simulink model "dynamic_8_edit"  (R2020b)
settings: Solver=ode5  StartTime=0.0  StopTime=60  FixedStep=0.1  RelTol=1e-3
libraries: simulink x2
settings Model: Creator=skets  LastModifiedBy=skets
settings SolverCC: ConcurrentTasks=on  PositivePriorityOrder=on
settings DataIOCC: ReturnWorkspaceOutputs=off
settings OptimizationCC: BlockReduction=off  DefaultParameterBehavior=Inlined  EnhancedBackFolding=on  PassReuseOutputArgsThreshold=0  OptimizeBlockOrder=speed  DifferentSizesBufferReuse=on  OptimizationCustomize=off
settings DebuggingCC: ParameterTunabilityLossMsg=error  ArithmeticOperatorsInVariantConditions=warning
settings SFSimCC: SimUseLocalCustomCode=off  MATLABDynamicMemAlloc=off  CustomCodeUndefinedFunction=UseInterfaceOnly
settings RTWCC: PackageGeneratedCodeAndArtifacts=on  PackageName=dynamic_circle  RTWUseLocalCustomCode=off  Toolchain=MinGW64 | gmake (64-bit Windows)  BuildConfiguration=Debug
settings CodeAppCC: ForceParamTrailComments=on  OperatorAnnotations=on

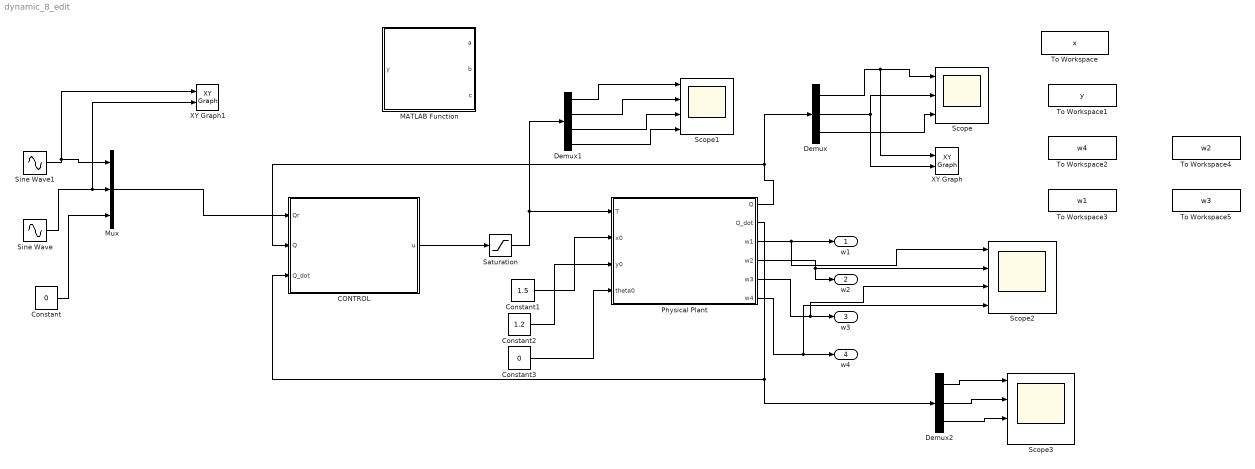
== system dynamic_8_edit ==
  CONTROL : Subsystem
  Constant : Constant  Value=0
  Constant1 : Constant  Value=1.5
  Constant2 : Constant  Value=1.2
  Constant3 : Constant  Value=0
  Demux : Demux  Outputs=3
  Demux1 : Demux
  Demux2 : Demux  Outputs=3
  MATLAB Function : MATLAB Function  TreatAsAtomicUnit=on
  Mux : Mux  Inputs=3
  Physical Plant : Subsystem
  Saturation : Saturate  UpperLimit=5  LowerLimit=-5
  Scope : Scope  NumInputPorts=3
  Scope1 : Scope  NumInputPorts=4
  Scope2 : Scope  NumInputPorts=4
  Scope3 : Scope  NumInputPorts=4
  Sine Wave : Sin  Bias=1.2  Frequency=4*pi/30
  Sine Wave1 : Sin  Bias=1.5  Frequency=2*pi/30
  To Workspace : ToWorkspace  VariableName=x  SampleTime=-1
  To Workspace1 : ToWorkspace  VariableName=y  SampleTime=-1
  To Workspace2 : ToWorkspace  VariableName=w4  SampleTime=-1
  To Workspace3 : ToWorkspace  VariableName=w1  SampleTime=-1
  To Workspace4 : ToWorkspace  VariableName=w2  SampleTime=-1
  To Workspace5 : ToWorkspace  VariableName=w3  SampleTime=-1
  XY Graph : simulink/Sinks/XY Graph  xmin=0  xmax=3  ymin=0  ymax=3  st=-1
  XY Graph1 : simulink/Sinks/XY Graph  xmin=0  xmax=2  ymin=0  ymax=2  st=-1
  w1 : Outport  VectorParamsAs1DForOutWhenUnconnected=off
  w2 : Outport  Port=2  VectorParamsAs1DForOutWhenUnconnected=off
  w3 : Outport  Port=3  VectorParamsAs1DForOutWhenUnconnected=off
  w4 : Outport  Port=4  VectorParamsAs1DForOutWhenUnconnected=off
  wires:
  Sine Wave/1 -> XY Graph1/2, Mux/2
  Constant/1 -> Mux/3
  Sine Wave1/1 -> XY Graph1/1, Mux/1
  Mux/1 -> CONTROL/1(Qr)
  CONTROL/1(u) -> Saturation/1
  Saturation/1 -> Demux1/1, Physical Plant/1(T)
  Physical Plant/3(w1) -> Scope2/1, w1/1
  Physical Plant/4(w2) -> Scope2/2, w2/1
  Physical Plant/5(w3) -> Scope2/3, w3/1
  Demux/1 -> XY Graph/1, Scope/1
  Demux/2 -> Scope/2, XY Graph/2
  Demux/3 -> Scope/3
  Demux1/1 -> Scope1/1
  Demux1/2 -> Scope1/2
  Demux1/3 -> Scope1/3
  Demux1/4 -> Scope1/4
  Physical Plant/2(Q_dot) -> CONTROL/3(Q_dot), Demux2/1
  Demux2/1 -> Scope3/1
  Demux2/2 -> Scope3/2
  Demux2/3 -> Scope3/3
  Constant1/1 -> Physical Plant/2(x0)
  Constant2/1 -> Physical Plant/3(y0)
  Constant3/1 -> Physical Plant/4(theta0)
  Physical Plant/6(w4) -> Scope2/4, w4/1
  Physical Plant/1(Q) -> CONTROL/2(Q), Demux/1

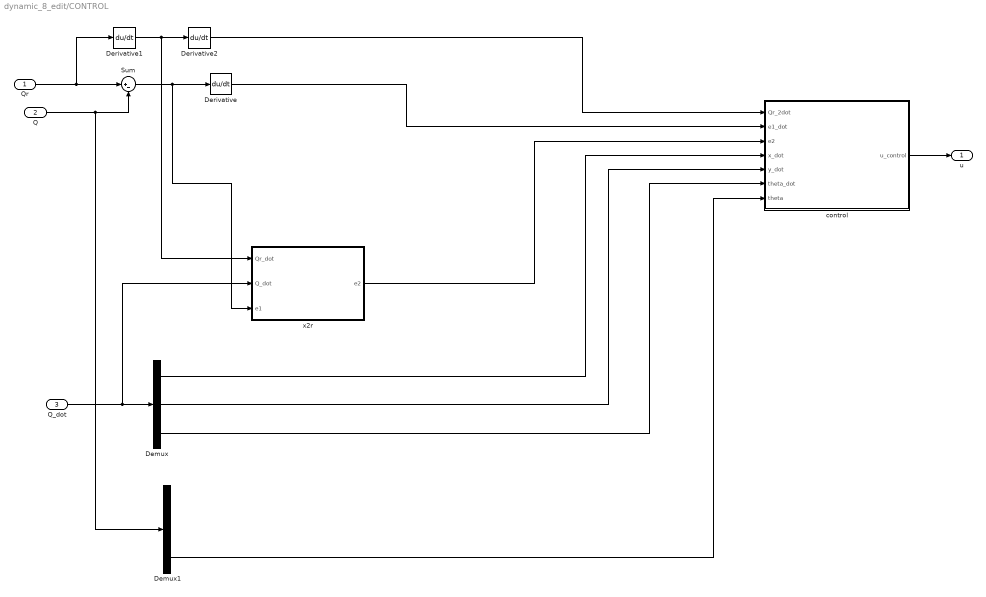
== system dynamic_8_edit/CONTROL ==
  Qr : Inport
  Q : Inport  Port=2  PortDimensions=3
  Q_dot : Inport  Port=3
  Demux : Demux  Outputs=3
  Demux1 : Demux  Outputs=3
  Derivative : Derivative
  Derivative1 : Derivative
  Derivative2 : Derivative
  Sum : Sum  Inputs=|+-
  control : MATLAB Function  TreatAsAtomicUnit=on
  x2r : MATLAB Function  TreatAsAtomicUnit=on
  u : Outport  VectorParamsAs1DForOutWhenUnconnected=off
  wires:
  Qr/1 -> Derivative1/1, Sum/1
  control/1(u_control) -> u/1
  Q/1 -> Demux1/1, Sum/2
  Demux/1 -> control/4(x_dot)
  Demux/2 -> control/5(y_dot)
  Demux/3 -> control/6(theta_dot)
  Demux1/3 -> control/7(theta)
  Sum/1 -> x2r/3(e1), Derivative/1
  Derivative2/1 -> control/1(Qr_2dot)
  Derivative/1 -> control/2(e1_dot)
  x2r/1(e2) -> control/3(e2)
  Derivative1/1 -> x2r/1(Qr_dot), Derivative2/1
  Q_dot/1 -> x2r/2(Q_dot), Demux/1

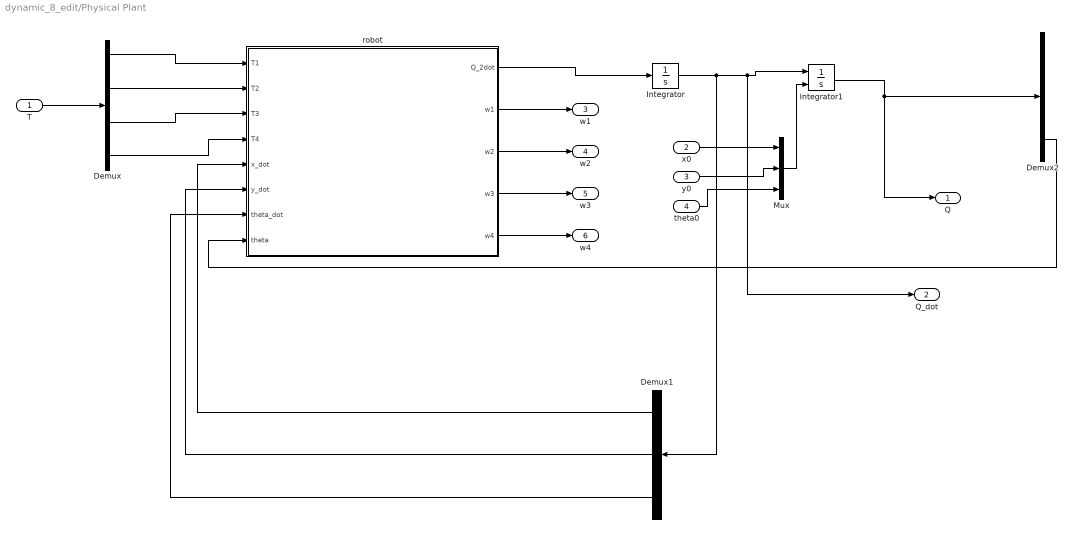
== system dynamic_8_edit/Physical Plant ==
  T : Inport  PortDimensions=4
  x0 : Inport  Port=2  PortDimensions=1
  y0 : Inport  Port=3  PortDimensions=1
  theta0 : Inport  Port=4  PortDimensions=1
  Demux : Demux
  Demux1 : Demux  Outputs=3
  Demux2 : Demux  Outputs=3
  Integrator : Integrator
  Integrator1 : Integrator  InitialConditionSource=external  InitialCondition=[0.5 1 0]
  Mux : Mux  Inputs=3
  robot : MATLAB Function  TreatAsAtomicUnit=on
  Q : Outport  VectorParamsAs1DForOutWhenUnconnected=off
  Q_dot : Outport  Port=2  VectorParamsAs1DForOutWhenUnconnected=off
  w1 : Outport  Port=3  VectorParamsAs1DForOutWhenUnconnected=off
  w2 : Outport  Port=4  VectorParamsAs1DForOutWhenUnconnected=off
  w3 : Outport  Port=5  VectorParamsAs1DForOutWhenUnconnected=off
  w4 : Outport  Port=6  VectorParamsAs1DForOutWhenUnconnected=off
  wires:
  Demux/1 -> robot/1(T1)
  Demux/2 -> robot/2(T2)
  Demux/3 -> robot/3(T3)
  Demux/4 -> robot/4(T4)
  robot/1(Q_2dot) -> Integrator/1
  Demux1/1 -> robot/5(x_dot)
  Demux1/2 -> robot/6(y_dot)
  Demux1/3 -> robot/7(theta_dot)
  Integrator1/1 -> Demux2/1, Q/1
  Demux2/3 -> robot/8(theta)
  T/1 -> Demux/1
  robot/2(w1) -> w1/1
  robot/3(w2) -> w2/1
  robot/4(w3) -> w3/1
  robot/5(w4) -> w4/1
  Integrator/1 -> Demux1/1, Integrator1/1, Q_dot/1
  Mux/1 -> Integrator1/2
  x0/1 -> Mux/1
  y0/1 -> Mux/2
  theta0/1 -> Mux/3

== matlab function dynamic_8_edit/Physical Plant/robot ==
  data: T1 input; Q_2dot output; T2 input; T3 input; T4 input; x_dot input; y_dot input; theta_dot input; theta input; w1 output; w2 output; w3 output; w4 output
function [Q_2dot,w1,w2,w3,w4]  = fcn(T1, T2, T3, T4,x_dot,y_dot,theta_dot,theta)

m=5;
I=5;
Ib=0.1;
l1= 0.3;
l2=0.3;
r=0.048;
g=9.8;
u=0.01;
N = m*g/4;
M=[(m+4*Ib/(r*r)) 0 0; 0 (m+4*Ib/(r*r)) 0; 0 0 (I+4*Ib*(l1+l2)*(l1+l2)/(r*r))];
C= [(m+4*Ib/(r*r))*y_dot*theta_dot;-(m+4*Ib/(r*r))*x_dot*theta_dot;0 ];
B=(1/r)*[(cos(theta)+sin(theta)) (cos(theta)-sin(theta)) (cos(theta)+sin(theta)) (cos(theta)-sin(theta));
         (-cos(theta)+sin(theta)) (cos(theta)+sin(theta)) (-cos(theta)+sin(theta)) (cos(theta)+sin(theta)); 
         (-(l1+l2)) (l1+l2) (l1+l2) (-(l1+l2)) ];
T=[T1;T2;T3;T4];
xm= cos(theta)*x_dot+sin(theta)*y_dot;
ym= -sin(theta)*x_dot+cos(theta)*y_dot;
w1 = (1/r)*(xm-ym-(l1+l2)*theta_dot);
w2 = (1/r)*(xm+ym+(l1+l2)*theta_dot);
w3 = (1/r)*(xm-ym+(l1+l2)*theta_dot);
w4 = (1/r)*(xm+ym-(l1+l2)*theta_dot);
w_max = 2;
if w1 > w_max
    w1 = w_max; %w = 20.83
elseif w1 < -w_max
    w1 = -w_max;
end
if w2 > w_max
    w2 = w_max;
elseif w2 < -w_max
    w2 = -w_max;
end
if w3 > w_max
    w3 = w_max;
elseif w3 < -w_max
    w3 = -w_max;
end
if w4 > w_max
    w4 = w_max;
elseif w4 < -w_max
    w4 = -w_max;
end
Xi=[u*r*N*sign(w1);u*r*N*sign(w2);u*r*N*sign(w3);u*N*r*sign(w4)];

Q_2dot=inv(M)*(B*T-C-B*Xi);

== matlab function dynamic_8_edit/CONTROL/control ==
  data: Qr_2dot input; u_control output; e1_dot input; e2 input; x_dot input; y_dot input; theta_dot input; theta input
function u_control = fcn(Qr_2dot,e1_dot,e2,x_dot,y_dot,theta_dot,theta)

m=5;
I=5;
Ib=0.1;
l1= 0.3;
l2=0.3;
r=0.048;
g=9.8;
u=0.01;
N = m*g/4;
M=[(m+4*Ib/(r*r)) 0 0; 0 (m+4*Ib/(r*r)) 0; 0 0 (I+4*Ib*(l1+l2)*(l1+l2)/(r*r))];
C= [(m+4*Ib/(r*r))*y_dot*theta_dot;-(m+4*Ib/(r*r))*x_dot*theta_dot;0 ];
B=(1/r)*[(cos(theta)+sin(theta)) (cos(theta)-sin(theta)) (cos(theta)+sin(theta)) (cos(theta)-sin(theta));
    (-cos(theta)+sin(theta)) (cos(theta)+sin(theta)) (-cos(theta)+sin(theta)) (cos(theta)+sin(theta)); 
    (-(l1+l2)) (l1+l2) (l1+l2) (-(l1+l2)) ];

xm= cos(theta)*x_dot+sin(theta)*y_dot;
ym= -sin(theta)*x_dot+cos(theta)*y_dot;
w1 = (1/r)*(xm-ym-(l1+l2)*theta_dot);
w2 = (1/r)*(xm+ym+(l1+l2)*theta_dot);
w3 = (1/r)*(xm-ym+(l1+l2)*theta_dot);
w4 = (1/r)*(xm+ym-(l1+l2)*theta_dot);
w_max = 2;

if w1 > w_max
    w1 = w_max; %w = 20.83
elseif w1 < -w_max
    w1 = -w_max;
end
if w2 > w_max
    w2 = w_max;
elseif w2 < -w_max
    w2 = -w_max;
end
if w3 > w_max
    w3 = w_max;
elseif w3 < -w_max
    w3 = -w_max;
end
if w4 > w_max
    w4 = w_max;
elseif w4 < -w_max
    w4 = -w_max;
end
Xi=[u*r*N*sign(w1);u*r*N*sign(w2);u*r*N*sign(w3);u*N*r*sign(w4)];

k1 = [0.5 0 0;
      0 0.5 0;
      0 0 0.5];
k2 = [0.5 0 0;
      0 0.5 0;
      0 0 0.5];
  
u_control = B'*inv(B*B')*M*((Qr_2dot+k1*e1_dot)+inv(M)*C+inv(M)*B*Xi+k2*e2);

== matlab function dynamic_8_edit/CONTROL/x2r ==
  data: Qr_dot input; Q_dot input; e2 output; e1 input
function e2  = fcn(Qr_dot,Q_dot,e1)

k1 = [0.5 0 0;
      0 0.5 0;
      0 0 0.5];
 
%x2r_dot = (Qr_2dot+k1*e1_dot);
x2r = Qr_dot + k1*e1;
e2 = x2r - Q_dot;

== matlab function dynamic_8_edit/MATLAB Function ==
  data: a input; y output; b input; c input
function y = fcn(a,b,c)
a =floor(a * 100) / 100;
b =floor(b * 100) / 100;
c =floor(c * 100) / 100;
y = [a; b; c];
